simulink model "Simulink_deel_1"  (R2016b)
settings: Solver=FixedStepAuto  StartTime=0.0  StopTime=100.0  FixedStep=0.001  RelTol=1e-3
settings Model: Creator=User  LastModifiedBy=User

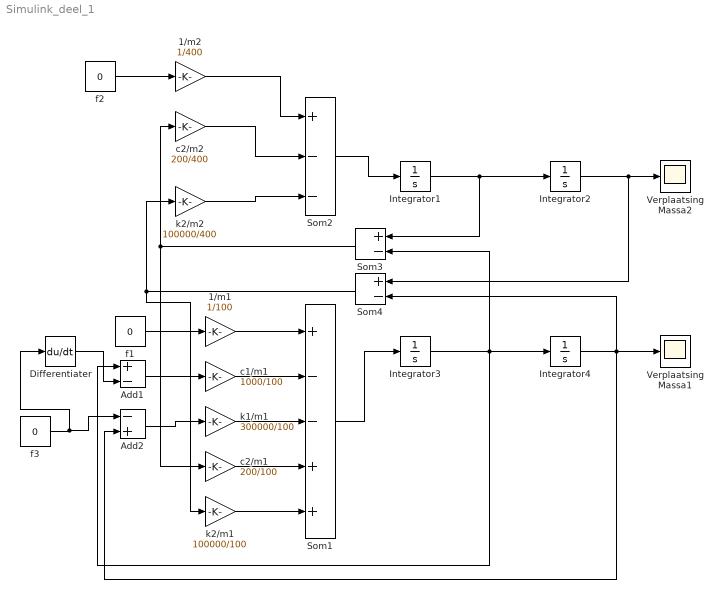
== system Simulink_deel_1 ==
  1/m1 : Gain  Gain=1/100
  1/m2 : Gain  Gain=1/400
  Add1 : Sum  Inputs=+-
  Add2 : Sum  Inputs=-+
  Differentiater : Derivative
  Integrator1 : Integrator
  Integrator2 : Integrator  InitialCondition=0.1
  Integrator3 : Integrator
  Integrator4 : Integrator
  Som1 : Sum  Inputs=+--++
  Som2 : Sum  Inputs=+--
  Som3 : Sum  Inputs=+-
  Som4 : Sum  Inputs=+-
  Verplaatsing Massa1 : Scope
  Verplaatsing Massa2 : Scope
  c1/m1 : Gain  Gain=1000/100
  c2/m1 : Gain  Gain=200/100
  c2/m2 : Gain  Gain=200/400
  f1 : Constant  Value=0
  f2 : Constant  Value=0
  f3 : Constant  Value=0
  k1/m1 : Gain  Gain=300000/100
  k2/m1 : Gain  Gain=100000/100
  k2/m2 : Gain  Gain=100000/400
  wires:
  Integrator1/1 -> Som3/1, Integrator2/1
  Integrator2/1 -> Som4/1, Verplaatsing Massa2/1
  Som2/1 -> Integrator1/1
  c2/m2/1 -> Som2/2
  k2/m2/1 -> Som2/3
  1/m2/1 -> Som2/1
  f2/1 -> 1/m2/1
  Som3/1 -> c2/m1/1, c2/m2/1
  Integrator4/1 -> Add2/2, Som4/2, Verplaatsing Massa1/1
  Som1/1 -> Integrator3/1
  Integrator3/1 -> Add1/1, Som3/2, Integrator4/1
  k2/m1/1 -> Som1/5
  c2/m1/1 -> Som1/4
  k1/m1/1 -> Som1/3
  c1/m1/1 -> Som1/2
  1/m1/1 -> Som1/1
  f1/1 -> 1/m1/1
  Add1/1 -> c1/m1/1
  Add2/1 -> k1/m1/1
  Differentiater/1 -> Add1/2
  f3/1 -> Add2/1, Differentiater/1
  Som4/1 -> k2/m1/1, k2/m2/1
